simulink model "flightSimulator"  (R2022a)
settings: Solver=VariableStepAuto  StartTime=0.0  StopTime=10.0  RelTol=1e-3
values from neighbouring files (symbols this model uses):
  g = 9.81    [LQRCalcs.m]    (also in cf_firstOrderStateMdl.m; init_parameters.m; main.m; parameters_buildingSimulink.m)
  Gamma = [cT, cT, cT, cT ... (first row only)    [init_parameters.m]    (also in parameters_buildingSimulink.m; parameters_init.m; parameters_init2.m; parameters_init____CodeToImplementLater.m)
  GammaInv = inv(Gamma)    [init_parameters.m]    (also in parameters_buildingSimulink.m; parameters_init.m; parameters_init2.m)
  J = cat(2, [0 0 0]', J)    [LQRCalcs.m]    (also in init_parameters.m = diag([0.082, 0.0845, 0.1377]); main.m = diag([0.082, 0.0845, 0.1377]); parameters_buildingSimulink.m = diag([0.082, 0.0845, 0.1377]); parameters_init.m = Crazyflie.J)
  k_motors = 1    [parameters_buildingSimulink.m]
  k_R = 8.81    [init_parameters.m]    (also in parameters_init____CodeToImplementLater.m)
  Kd_attitude = 0.01    [parameters_buildingSimulink.m]
  Kd_eta = 0    [init_parameters.m]
  Kp_attitude = 0.5    [parameters_buildingSimulink.m]
  Kp_eta = 0    [init_parameters.m]
  m = 0.003    [LQRCalcs.m]    (also in cf_firstOrderStateMdl.m; init_parameters.m = 4.34; main.m = 4.34; parameters_buildingSimulink.m = 4.34)
  XYZ_initial_condition = [0, 0, 0]'    [init_parameters.m]
undefined symbols (not defined in the file or in its folder): k_Omega
libraries: slpidlib x2, aerolibutil x2
settings Model: Creator=Drew Lab Computer 1  LastModifiedBy=Drew Lab Computer 1

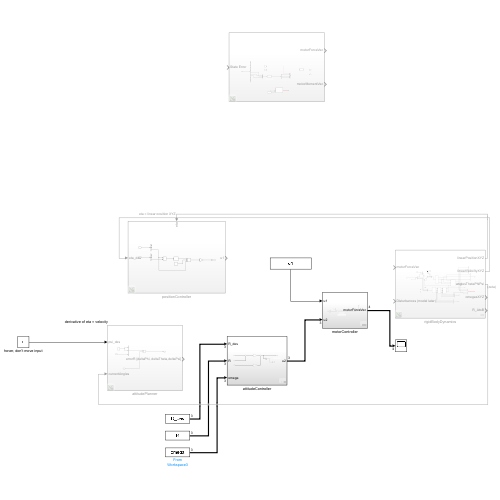
[thumbnail: Simulink's stored preview of the top-level diagram]
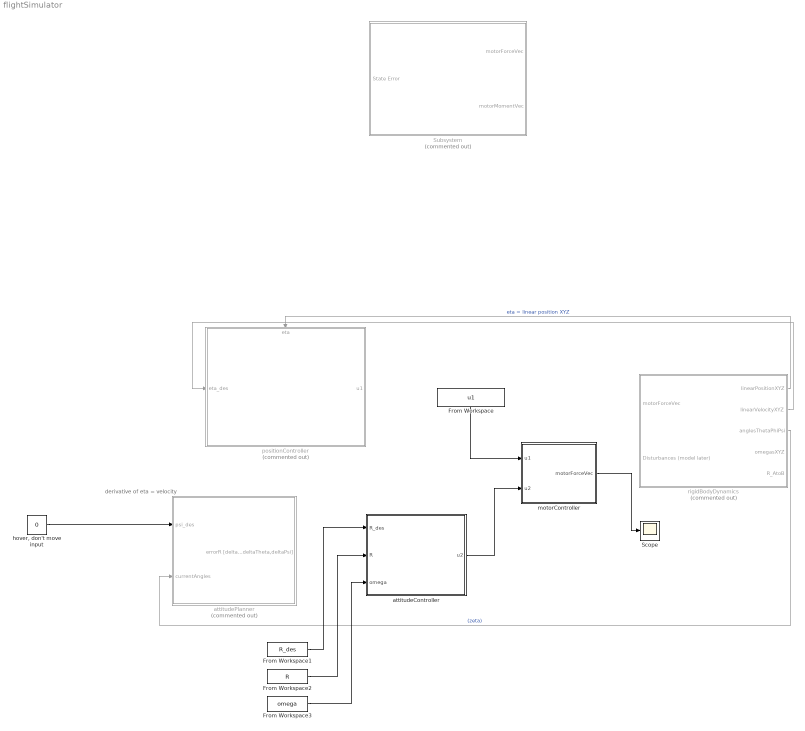
== system flightSimulator ==
  note: derivative of eta = velocity
  From Workspace : FromWorkspace  VariableName=u1
  From Workspace1 : FromWorkspace  VariableName=R_des
  From Workspace2 : FromWorkspace  VariableName=R
  From Workspace3 : FromWorkspace  VariableName=omega
  Scope : Scope
  Subsystem : Subsystem  Commented=on
  attitudeController : Subsystem
  attitudePlanner : Subsystem  Commented=on
  "hover, don't move input" : Constant  Value=0
  motorController : Subsystem
  positionController : Subsystem  Commented=on
      settings: PortSchema="{\"entries\":[{\"content\":{\"sides\":[{\"content\":{\"connectorIds\":[\"In1\"]},\"type\":\"ConnectorPlacement.EquallySpacedRectSide\",\"uuid\":\"de936069-44f0-4aa9-b4b1-7b3705576372\"},{\"content\":{\"connectorIds\":[\"Out1\"],\"side\":\"RIGHT\"},\"type\":\"ConnectorPlacement.EquallySpacedRectSide\",\"uuid\":\"f2caec36-291a-4389-af1f-a91b49b87c15\"},{\"content\":{\"connectorIds\":[\"In2\"],\"side\":\"TOP\"},\"type\":\"ConnectorPlacement.EquallySpacedRectSide\",\"uuid\":\"cd074ac1-2f19-4ea9-a351-803ac25dc689\"}]},\"type\":\"ConnectorPlacement.EquallySpacedConnector\",\"uuid\":\"58e30618-1523-4ed1-9bdc-0936c58338cb\"}],\"packageUris\":[\"http://schema.mathworks.com/mf0/Connector/R2020b\"],\"version\":\"1.0\"}"
  rigidBodyDynamics : Subsystem  Commented=on
  wires:
  rigidBodyDynamics/1(linearPositionXYZ) -> positionController/2(eta)  "eta = linear position XYZ"
  rigidBodyDynamics/3(anglesThetaPhiPsi) -> attitudePlanner/2(currentAngles)  "(zeta)"
  "hover, don't move input"/1 -> attitudePlanner/1(psi_des)
  rigidBodyDynamics/2(linearVelocityXYZ) -> positionController/1(eta_des)
  attitudeController/1(u2) -> motorController/2(u2)
  From Workspace/1 -> motorController/1(u1)
  From Workspace1/1 -> attitudeController/1(R_des)
  From Workspace2/1 -> attitudeController/2(R)
  From Workspace3/1 -> attitudeController/3(omega)
  motorController/1(motorForceVec) -> Scope/1

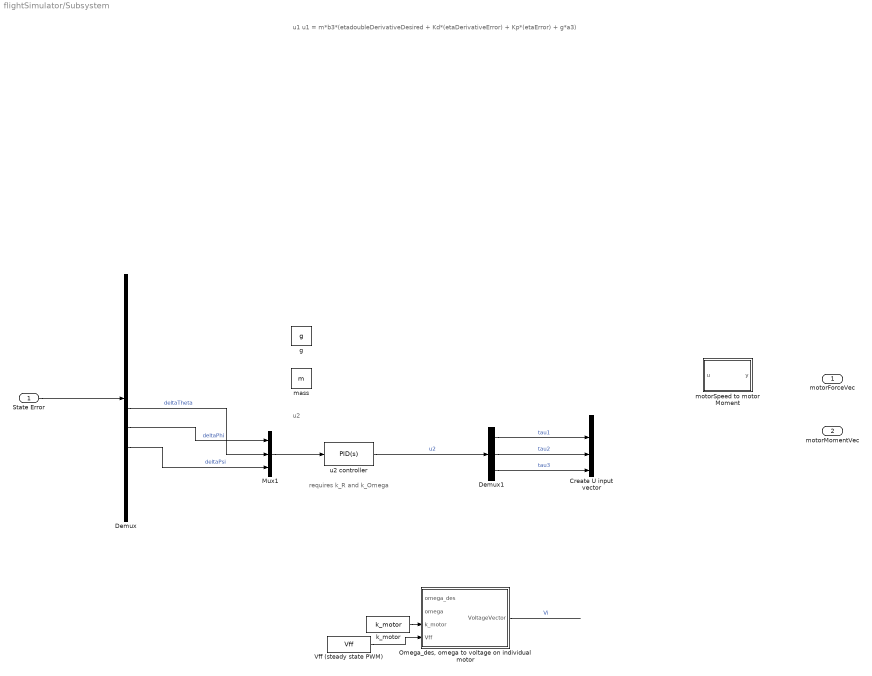
== system flightSimulator/Subsystem ==
  note: requires k_R and k_Omega
  note: u2
  note: u1
      | u1 = m*b3*(etadoubleDerivativeDesired + Kd*(etaDerivativeError) + Kp*(etaError) + g*a3)
  State Error : Inport
  Create U input vector : Mux
  Demux : Demux  Outputs=12
  Demux1 : Demux  Outputs=3
  Mux1 : Mux  Inputs=3
  "Omega_des, omega to voltage on individual motor" : MATLAB Function  TreatAsAtomicUnit=on
  Vff (steady state PWM) : FromWorkspace  VariableName=Vff
  g : Constant  Value=g
  k_motor : FromWorkspace  VariableName=k_motor
  mass : Constant  Value=m
  motorSpeed to motor Moment : MATLAB Function  TreatAsAtomicUnit=on
  u2 controller : slpidlib/PID Controller  Controller=PID  Form=Parallel  TimeDomain=Continuous-time  UseExternalTs=off  SampleTime=-1  IntegratorMethod=Forward Euler  FilterMethod=Forward Euler  ControllerParametersSource=internal  P=k_R  I=1  UseKiTs=off  D=k_Omega  N=100  UseFilter=on  TunerSelectOption=Transfer Function Based (PID Tuner App)  InitialConditionSource=internal  InitialConditionForIntegrator=0  InitialConditionForFilter=0  DifferentiatorICPrevScaledInput=0  ExternalReset=none  TrackingMode=off  Kt=1  LimitOutput=off  SatLimitsSource=internal  UpperSaturationLimit=inf  LowerSaturationLimit=-inf  LinearizeAsGain=on  AntiWindupMode=none  Kb=1  POutMin=[]  POutMax=[]  IOutMin=[]  IOutMax=[]  DOutMin=[]  DOutMax=[]  NOutMin=[]  NOutMax=[]  SumOutMin=[]  SumOutMax=[]  SaturationOutMin=[]  SaturationOutMax=[]  PParamMin=[]  PParamMax=[]  IParamMin=[]  IParamMax=[]  DParamMin=[]  DParamMax=[]  NParamMin=[]  NParamMax=[]  KbParamMin=[]  KbParamMax=[]  KtParamMin=[]  KtParamMax=[]  KbOutMin=[]  KbOutMax=[]  KtOutMin=[]  KtOutMax=[]  IntegratorOutMin=[]  IntegratorOutMax=[]  FilterOutMin=[]  FilterOutMax=[]  SumI1OutMin=[]  SumI1OutMax=[]  SumI2OutMin=[]  SumI2OutMax=[]  SumI3OutMin=[]  SumI3OutMax=[]  SumI4OutMin=[]  SumI4OutMax=[]  SumDOutMin=[]  SumDOutMax=[]  DifferentiatorOutMin=[]  DifferentiatorOutMax=[]  FilterDiffOutCoefMin=[]  FilterDiffOutCoefMax=[]  ReciprocalOutMin=[]  ReciprocalOutMax=[]  SumDenOutMin=[]  SumDenOutMax=[]  SumNumOutMin=[]  SumNumOutMax=[]  DivideOutMin=[]  DivideOutMax=[]  UdiffTsProdOutMin=[]  UdiffTsProdOutMax=[]  NTsProdOutMin=[]  NTsProdOutMax=[]  UintegralTsProdOutMin=[]  UintegralTsProdOutMax=[]  UngainTsProdOutMin=[]  UngainTsProdOutMax=[]  IntegratorContinuousStateAttributes=''  IntegratorStateMustResolveToSignalObject=off  IntegratorRTWStateStorageClass=Auto  FilterContinuousStateAttributes=''  FilterStateMustResolveToSignalObject=off  FilterRTWStateStorageClass=Auto  ParallelPVariant=InternalParameters  IdealPVariant=Disabled  IVariant=InternalParameters  DVariant=InternalParameters  IntegratorVariant=Continuous  SatVariant=Disabled  AWVariant=Passthrough  PCopyVariant=Disabled  TRVariant=Disabled  FdbkBlocksVariant=Forward  IdealPFdbkVariant=Disabled  SatFdbkVariant=Disabled  DerivativeFilterVariant=ContFilter  NVariant=InternalParameters  NCopyVariant=Disabled  FilterICVariant=InternalICsFilter  IntegratorICVariant=InternalICs  ExternalResetVariant=Disabled  TRSumVariant=Passthrough  SumFdbkVariant=Disabled  SumVariant=Sum_PID  TsampFilterVariant=InternalTs  TsampNgainVariant=Passthrough  TsampIntegralVariant=Passthrough  ExternalSaturationOutDataTypeStr=Inherit: Same as second input  aMode=0
  motorForceVec : Outport
  motorMomentVec : Outport  Port=2
  wires:
  "Omega_des, omega to voltage on individual motor"/1(VoltageVector) -> ?  "Vi"
  State Error/1 -> Demux/1
  Demux/8 -> Mux1/1  "deltaPhi"
  Demux/9 -> Mux1/3  "deltaPsi"
  k_motor/1 -> "Omega_des, omega to voltage on individual motor"/3(k_motor)
  Vff (steady state PWM)/1 -> "Omega_des, omega to voltage on individual motor"/4(Vff)
  Demux/7 -> Mux1/2  "deltaTheta"
  Mux1/1 -> u2 controller/1
  u2 controller/1 -> Demux1/1  "u2"
  ? -> Create U input vector/1  "thrustSum"
  Demux1/3 -> Create U input vector/4  "tau3"
  Demux1/2 -> Create U input vector/3  "tau2"
  Demux1/1 -> Create U input vector/2  "tau1"

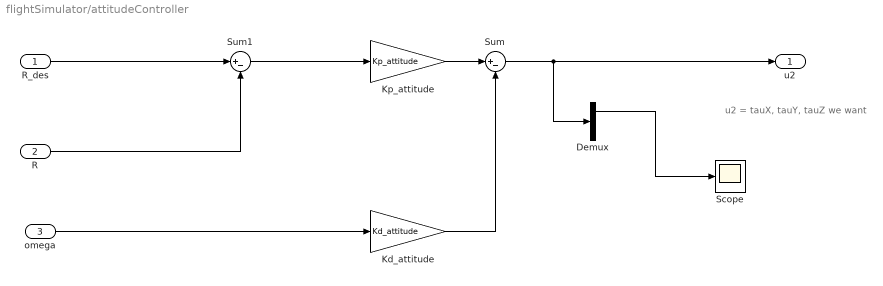
== system flightSimulator/attitudeController ==
  note: u2 = tauX, tauY, tauZ we want
  R_des : Inport
  R : Inport  Port=2
  omega : Inport  Port=3
  Demux : Demux  Outputs=3
  Kd_attitude : Gain  Gain=Kd_attitude
  Kp_attitude : Gain  Gain=Kp_attitude
  Scope : Scope
  Sum : Sum  Inputs=|+-
  Sum1 : Sum  Inputs=|+-
  u2 : Outport
  wires:
  Kp_attitude/1 -> Sum/1
  Kd_attitude/1 -> Sum/2
  Sum/1 -> Demux/1, u2/1
  R_des/1 -> Sum1/1
  R/1 -> Sum1/2
  Sum1/1 -> Kp_attitude/1
  omega/1 -> Kd_attitude/1
  Demux/1 -> Scope/1

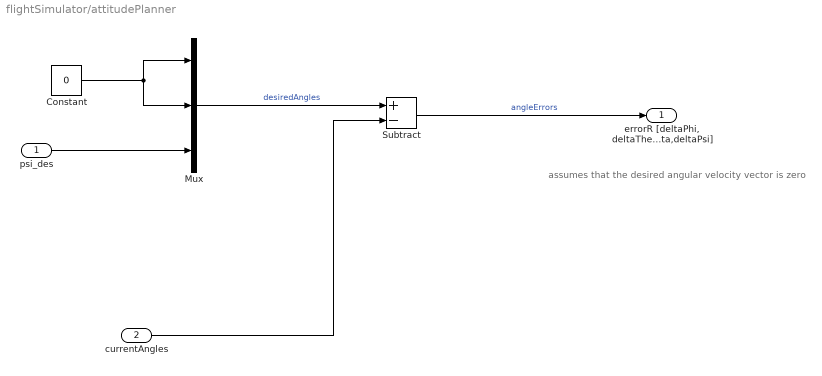
== system flightSimulator/attitudePlanner ==
  note: assumes that the desired angular velocity vector is zero
  psi_des : Inport
  currentAngles : Inport  Port=2
  Constant : Constant  Value=0
  Mux : Mux  Inputs=3
  Subtract : Sum  Inputs=+-
  "errorR [deltaPhi, deltaTheta,deltaPsi]" : Outport
  wires:
  psi_des/1 -> Mux/3
  Constant/1 -> Mux/1, Mux/2
  Mux/1 -> Subtract/1  "desiredAngles"
  Subtract/1 -> "errorR [deltaPhi, deltaTheta,deltaPsi]"/1  "angleErrors"
  currentAngles/1 -> Subtract/2

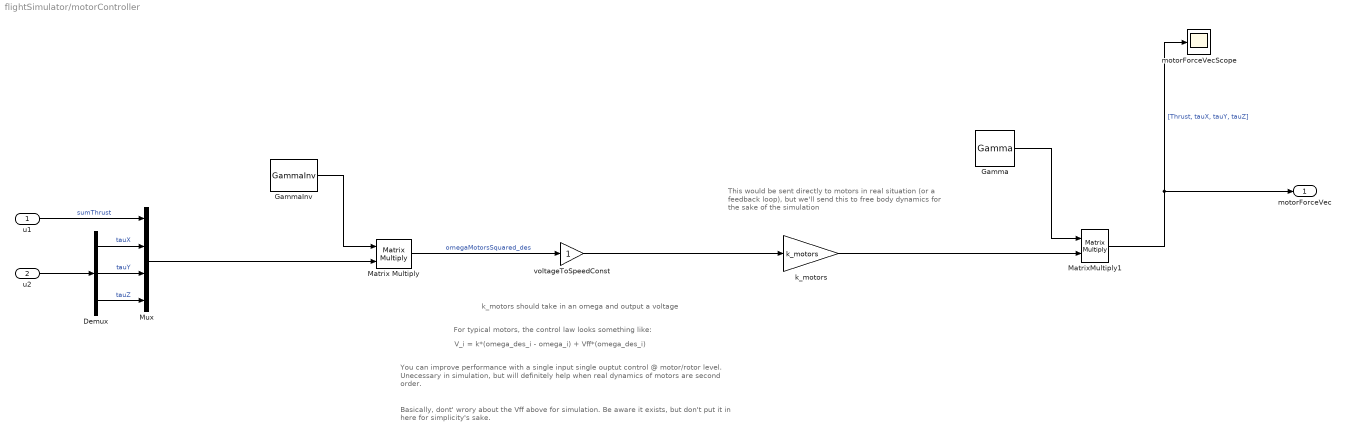
== system flightSimulator/motorController ==
  note: This would be sent directly to motors in real situation (or a feedback loop), but we'll send this to free body dynamics for the sake of the simulation
  note: k_motors should take in an omega and output a voltage
  note: Basically, dont' wrory about the Vff above for simulation. Be aware it exists, but don't put it in here for simplicity's sake.
  note: You can improve performance with a single input single ouptut control @ motor/rotor level. Unecessary in simulation, but will definitely help when real dynamics of motors are second order.
  note: V_i = k*(omega_des_i - omega_i) + Vff*(omega_des_i)
  note: For typical motors, the control law looks something like:
  u1 : Inport
  u2 : Inport  Port=2
  Demux : Demux  Outputs=3
  Gamma : Constant  Value=Gamma
  GammaInv : Constant  Value=GammaInv
  Matrix Multiply : Product  Multiplication=Matrix(*)
  MatrixMultiply1 : Product  Multiplication=Matrix(*)
  Mux : Mux
  k_motors : Gain  Gain=k_motors
  motorForceVecScope : Scope
  voltageToSpeedConst : Gain
  motorForceVec : Outport
  wires:
  u2/1 -> Demux/1
  u1/1 -> Mux/1  "sumThrust"
  Demux/2 -> Mux/3  "tauY"
  Demux/1 -> Mux/2  "tauX"
  Demux/3 -> Mux/4  "tauZ"
  Gamma/1 -> MatrixMultiply1/1
  MatrixMultiply1/1 -> motorForceVec/1, motorForceVecScope/1  "[Thrust, tauX, tauY, tauZ]"
  Mux/1 -> Matrix Multiply/2
  GammaInv/1 -> Matrix Multiply/1
  Matrix Multiply/1 -> voltageToSpeedConst/1  "omegaMotorsSquared_des"
  voltageToSpeedConst/1 -> k_motors/1
  k_motors/1 -> MatrixMultiply1/2

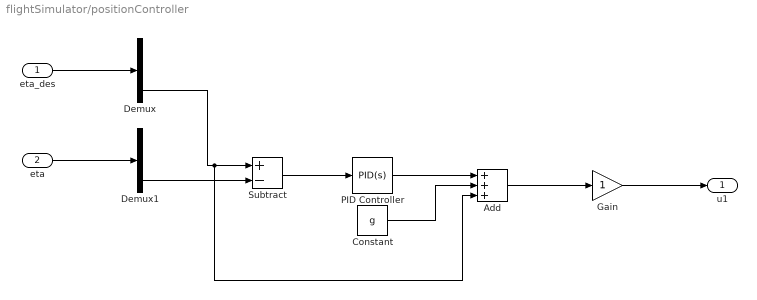
== system flightSimulator/positionController ==
  eta_des : Inport
  eta : Inport  Port=2
  Add : Sum  Inputs=+++
  Constant : Constant  Value=g
  Demux : Demux  Outputs=3
  Demux1 : Demux  Outputs=3
  Gain : Gain
  PID Controller : slpidlib/PID Controller  Controller=PID  Form=Parallel  TimeDomain=Continuous-time  UseExternalTs=off  SampleTime=-1  IntegratorMethod=Forward Euler  FilterMethod=Forward Euler  ControllerParametersSource=internal  P=Kp_eta  I=1  UseKiTs=off  D=Kd_eta  N=100  UseFilter=on  TunerSelectOption=Transfer Function Based (PID Tuner App)  InitialConditionSource=internal  InitialConditionForIntegrator=0  InitialConditionForFilter=0  DifferentiatorICPrevScaledInput=0  ExternalReset=none  TrackingMode=off  Kt=1  LimitOutput=off  SatLimitsSource=internal  UpperSaturationLimit=inf  LowerSaturationLimit=-inf  LinearizeAsGain=on  AntiWindupMode=none  Kb=1  POutMin=[]  POutMax=[]  IOutMin=[]  IOutMax=[]  DOutMin=[]  DOutMax=[]  NOutMin=[]  NOutMax=[]  SumOutMin=[]  SumOutMax=[]  SaturationOutMin=[]  SaturationOutMax=[]  PParamMin=[]  PParamMax=[]  IParamMin=[]  IParamMax=[]  DParamMin=[]  DParamMax=[]  NParamMin=[]  NParamMax=[]  KbParamMin=[]  KbParamMax=[]  KtParamMin=[]  KtParamMax=[]  KbOutMin=[]  KbOutMax=[]  KtOutMin=[]  KtOutMax=[]  IntegratorOutMin=[]  IntegratorOutMax=[]  FilterOutMin=[]  FilterOutMax=[]  SumI1OutMin=[]  SumI1OutMax=[]  SumI2OutMin=[]  SumI2OutMax=[]  SumI3OutMin=[]  SumI3OutMax=[]  SumI4OutMin=[]  SumI4OutMax=[]  SumDOutMin=[]  SumDOutMax=[]  DifferentiatorOutMin=[]  DifferentiatorOutMax=[]  FilterDiffOutCoefMin=[]  FilterDiffOutCoefMax=[]  ReciprocalOutMin=[]  ReciprocalOutMax=[]  SumDenOutMin=[]  SumDenOutMax=[]  SumNumOutMin=[]  SumNumOutMax=[]  DivideOutMin=[]  DivideOutMax=[]  UdiffTsProdOutMin=[]  UdiffTsProdOutMax=[]  NTsProdOutMin=[]  NTsProdOutMax=[]  UintegralTsProdOutMin=[]  UintegralTsProdOutMax=[]  UngainTsProdOutMin=[]  UngainTsProdOutMax=[]  IntegratorContinuousStateAttributes=''  IntegratorStateMustResolveToSignalObject=off  IntegratorRTWStateStorageClass=Auto  FilterContinuousStateAttributes=''  FilterStateMustResolveToSignalObject=off  FilterRTWStateStorageClass=Auto  ParallelPVariant=InternalParameters  IdealPVariant=Disabled  IVariant=InternalParameters  DVariant=InternalParameters  IntegratorVariant=Continuous  SatVariant=Disabled  AWVariant=Passthrough  PCopyVariant=Disabled  TRVariant=Disabled  FdbkBlocksVariant=Forward  IdealPFdbkVariant=Disabled  SatFdbkVariant=Disabled  DerivativeFilterVariant=ContFilter  NVariant=InternalParameters  NCopyVariant=Disabled  FilterICVariant=InternalICsFilter  IntegratorICVariant=InternalICs  ExternalResetVariant=Disabled  TRSumVariant=Passthrough  SumFdbkVariant=Disabled  SumVariant=Sum_PID  TsampFilterVariant=InternalTs  TsampNgainVariant=Passthrough  TsampIntegralVariant=Passthrough  ExternalSaturationOutDataTypeStr=Inherit: Same as second input  aMode=0
  Subtract : Sum  Inputs=+-
  u1 : Outport
  wires:
  eta_des/1 -> Demux/1
  Subtract/1 -> PID Controller/1
  eta/1 -> Demux1/1
  Demux/3 -> Add/3, Subtract/1
  Demux1/3 -> Subtract/2
  PID Controller/1 -> Add/1
  Constant/1 -> Add/2
  Add/1 -> Gain/1
  Gain/1 -> u1/1

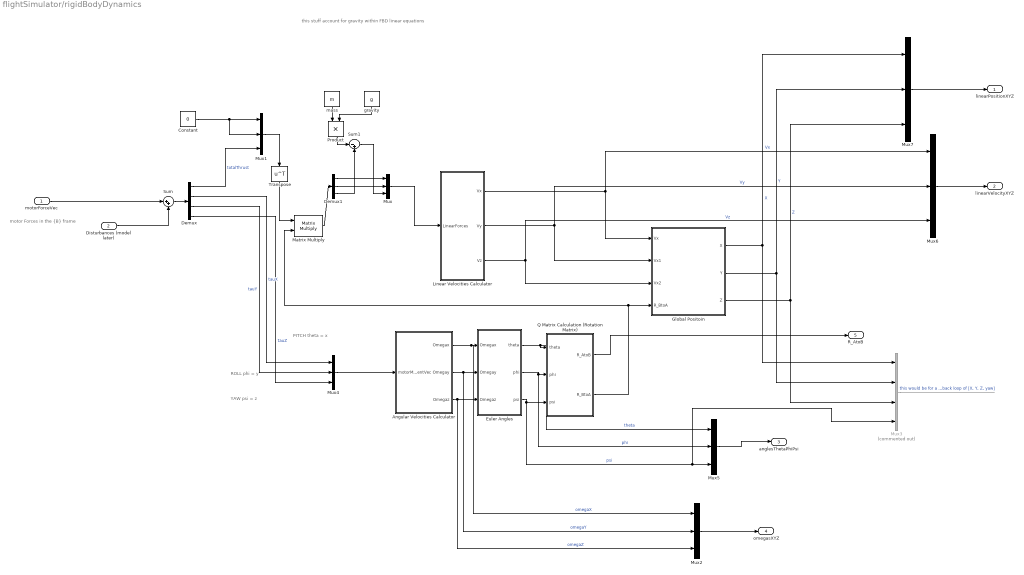
== system flightSimulator/rigidBodyDynamics ==
  note: YAW
      | psi = z
  note: ROLL
      | phi = y
  note: PITCH
      | theta = x
  note: this stuff account for gravity within FBD linear equations
  note: motor Forces in the {B} frame
  motorForceVec : Inport
  Disturbances (model later) : Inport  Port=2
  Angular Velocities Calculator : Subsystem
  Constant : Constant  Value=0
  Demux : Demux
  Demux1 : Demux  Outputs=3
  Euler Angles : Subsystem
  Global Positoin : Subsystem
  Linear Velocities Calculator : Subsystem
  Matrix Multiply : Product  Multiplication=Matrix(*)
  Mux{,1..2,4..7} (7 alike) : Mux  Inputs=3
  Mux3 : Mux  Commented=on
  Product : Product
  Q Matrix Calculation (Rotation Matrix) : Subsystem
  Sum : Sum  Inputs=|++
  Sum1 : Sum  Inputs=|-+
  Transpose : Math  Operator=transpose
  gravity : Constant  Value=g
  mass : Constant  Value=m
  linearPositionXYZ : Outport
  linearVelocityXYZ : Outport  Port=2
  anglesThetaPhiPsi : Outport  Port=3
  omegasXYZ : Outport  Port=4
  R_AtoB : Outport  Port=5
  wires:
  Transpose/1 -> Matrix Multiply/1
  Mux1/1 -> Transpose/1
  motorForceVec/1 -> Sum/1
  Disturbances (model later)/1 -> Sum/2
  Linear Velocities Calculator/1(Vx) -> Mux6/1, Global Positoin/1(Vx)  "Vx"
  Linear Velocities Calculator/2(Vy) -> Mux6/2, Global Positoin/2(Vx1)  "Vy"
  Linear Velocities Calculator/3(Vz) -> Mux6/3, Global Positoin/3(Vx2)  "Vz"
  Q Matrix Calculation (Rotation Matrix)/2(R_BtoA) -> Matrix Multiply/2, Global Positoin/4(R_BtoA)
  Mux4/1 -> Angular Velocities Calculator/1(motorMomentVec)
  Angular Velocities Calculator/3(Omegaz) -> Mux2/3, Euler Angles/3(Omegaz)  "omegaZ"
  Angular Velocities Calculator/2(Omegay) -> Mux2/2, Euler Angles/2(Omegay)  "omegaY"
  Angular Velocities Calculator/1(Omegax) -> Mux2/1, Euler Angles/1(Omegax)  "omegaX"
  Euler Angles/2(phi) -> Mux5/2, Q Matrix Calculation (Rotation Matrix)/2(phi)  "phi"
  Euler Angles/1(theta) -> Mux5/1, Q Matrix Calculation (Rotation Matrix)/1(theta)  "theta"
  Euler Angles/3(psi) -> Mux3/4, Mux5/3, Q Matrix Calculation (Rotation Matrix)/3(psi)  "psi"
  Mux/1 -> Linear Velocities Calculator/1(LinearForces)
  Product/1 -> Sum1/1
  Sum1/1 -> Mux/3
  mass/1 -> Product/1
  gravity/1 -> Product/2
  Global Positoin/3(Z) -> Mux7/3, Mux3/3  "Z"
  Global Positoin/2(Y) -> Mux7/2, Mux3/2  "Y"
  Global Positoin/1(X) -> Mux7/1, Mux3/1  "X"
  Mux3/1 -> ?  "this would be for a feedback loop of [X, Y, Z, yaw]"
  Sum/1 -> Demux/1
  Demux/1 -> Mux1/3  "totalThrust"
  Demux1/3 -> Sum1/2
  Demux1/2 -> Mux/2
  Demux1/1 -> Mux/1
  Demux/3 -> Mux4/2  "tauY"
  Demux/4 -> Mux4/3  "tauZ"
  Demux/2 -> Mux4/1  "tauX"
  Q Matrix Calculation (Rotation Matrix)/1(R_AtoB) -> R_AtoB/1
  Mux2/1 -> omegasXYZ/1
  Mux5/1 -> anglesThetaPhiPsi/1
  Mux7/1 -> linearPositionXYZ/1
  Mux6/1 -> linearVelocityXYZ/1
  Constant/1 -> Mux1/2, Mux1/1
  Matrix Multiply/1 -> Demux1/1

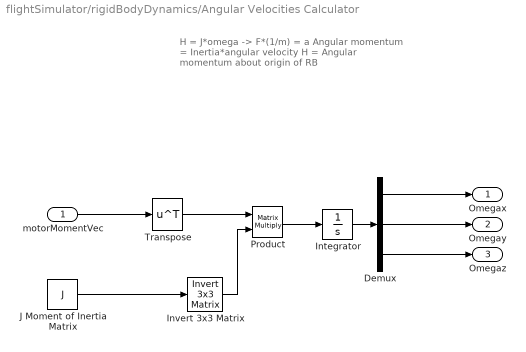
== system flightSimulator/rigidBodyDynamics/Angular Velocities Calculator ==
  note: H = J*omega -> F*(1/m) = a
      | Angular momentum = Inertia*angular velocity
      | H = Angular momentum about origin of RB
  motorMomentVec : Inport
  Demux : Demux  Outputs=3
  Integrator : Integrator
  Invert 3x3 Matrix : aerolibutil/Invert  3x3 Matrix
  J Moment of Inertia Matrix : Constant  Value=J
  Product : Product  Multiplication=Matrix(*)
  Transpose : Math  Operator=transpose
  Omegax : Outport
  Omegay : Outport  Port=2
  Omegaz : Outport  Port=3
  wires:
  Transpose/1 -> Product/1
  motorMomentVec/1 -> Transpose/1
  Demux/1 -> Omegax/1
  Demux/2 -> Omegay/1
  Demux/3 -> Omegaz/1
  Product/1 -> Integrator/1
  Integrator/1 -> Demux/1
  J Moment of Inertia Matrix/1 -> Invert 3x3 Matrix/1
  Invert 3x3 Matrix/1 -> Product/2

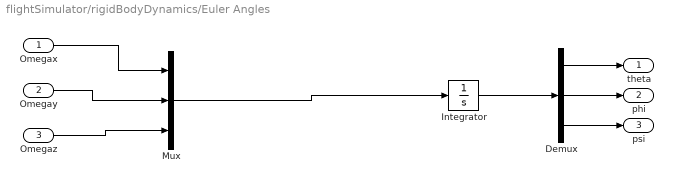
== system flightSimulator/rigidBodyDynamics/Euler Angles ==
  Omegax : Inport
  Omegay : Inport  Port=2
  Omegaz : Inport  Port=3
  Demux : Demux  Outputs=3
  Integrator : Integrator
  Mux : Mux  Inputs=3
  theta : Outport
  phi : Outport  Port=2
  psi : Outport  Port=3
  wires:
  Omegaz/1 -> Mux/3
  Omegay/1 -> Mux/2
  Omegax/1 -> Mux/1
  Integrator/1 -> Demux/1
  Demux/2 -> phi/1
  Demux/1 -> theta/1
  Demux/3 -> psi/1
  Mux/1 -> Integrator/1

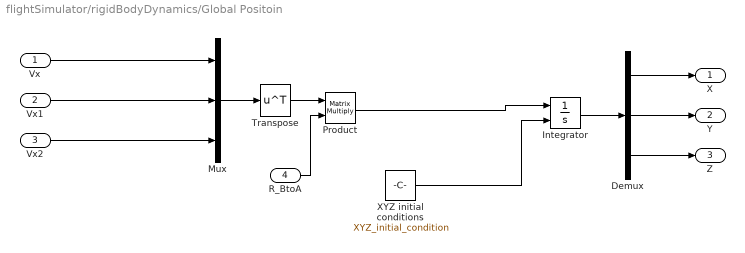
== system flightSimulator/rigidBodyDynamics/Global Positoin ==
  Vx : Inport
  Vx1 : Inport  Port=2
  Vx2 : Inport  Port=3
  R_BtoA : Inport  Port=4
  Demux : Demux  Outputs=3
  Integrator : Integrator  InitialConditionSource=external
  Mux : Mux  Inputs=3
  Product : Product  Multiplication=Matrix(*)
  Transpose : Math  Operator=transpose
  XYZ initial conditions : Constant  Value=XYZ_initial_condition
  X : Outport
  Y : Outport  Port=2
  Z : Outport  Port=3
  wires:
  Mux/1 -> Transpose/1
  Transpose/1 -> Product/1
  XYZ initial conditions/1 -> Integrator/2
  Product/1 -> Integrator/1
  Integrator/1 -> Demux/1
  Demux/2 -> Y/1
  Demux/1 -> X/1
  Demux/3 -> Z/1
  Vx2/1 -> Mux/3
  Vx1/1 -> Mux/2
  Vx/1 -> Mux/1
  R_BtoA/1 -> Product/2

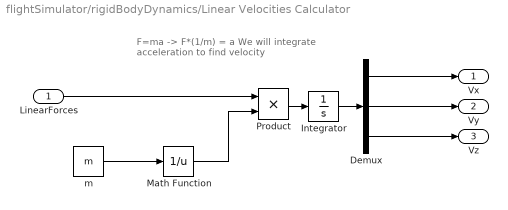
== system flightSimulator/rigidBodyDynamics/Linear Velocities Calculator ==
  note: F=ma -> F*(1/m) = a
      | We will integrate acceleration to find velocity
  LinearForces : Inport
  Demux : Demux  Outputs=3
  Integrator : Integrator
  Math Function : Math  Operator=reciprocal  SignedPower=on
  Product : Product
  m : Constant  Value=m
  Vx : Outport
  Vy : Outport  Port=2
  Vz : Outport  Port=3
  wires:
  LinearForces/1 -> Product/1
  m/1 -> Math Function/1
  Math Function/1 -> Product/2
  Demux/1 -> Vx/1
  Demux/2 -> Vy/1
  Demux/3 -> Vz/1
  Product/1 -> Integrator/1
  Integrator/1 -> Demux/1

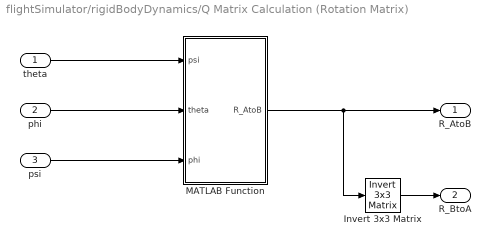
== system flightSimulator/rigidBodyDynamics/Q Matrix Calculation (Rotation Matrix) ==
  theta : Inport
  phi : Inport  Port=2
  psi : Inport  Port=3
  Invert 3x3 Matrix : aerolibutil/Invert  3x3 Matrix
  MATLAB Function : MATLAB Function  TreatAsAtomicUnit=on
  R_AtoB : Outport
  R_BtoA : Outport  Port=2
  wires:
  MATLAB Function/1(R_AtoB) -> Invert 3x3 Matrix/1, R_AtoB/1
  phi/1 -> MATLAB Function/2(theta)
  psi/1 -> MATLAB Function/3(phi)
  theta/1 -> MATLAB Function/1(psi)
  Invert 3x3 Matrix/1 -> R_BtoA/1

== matlab function flightSimulator/Subsystem/motorSpeed to motor Moment ==
  data: u input; y output
function y = fcn(u)

y = u;

== matlab function flightSimulator/rigidBodyDynamics/Q Matrix Calculation (Rotation Matrix)/MATLAB Function ==
  data: psi input; R_AtoB output; theta input; phi input
function R_AtoB = fcn(psi, theta, phi)

% R_AtoB = ...
%     [cos(psi)   -sin(psi) del_theta*cos(psi)+del_phi*sin(psi);
%      sin(psi),   cos(psi) del_theta*sin(psi)-del_phi*cos(psi);
%      -del_theta -del_phi 1;];

C_psi = cos(psi);
S_psi = sin(psi);
C_phi = cos(phi);
S_phi = sin(phi);
C_theta = cos(theta);
S_theta = sin(theta);
R_AtoB = ...
    [C_psi*C_theta-S_phi*S_psi*S_theta, -C_phi*S_phi, C_psi*S_theta+C_theta*S_phi*S_psi;
    C_theta*S_psi+C_psi*S_phi*S_theta, C_phi*C_psi, S_psi*S_theta-C_psi*C_theta*S_phi;
    -C_phi*S_theta, S_phi, C_phi*C_theta;];
%     [cos(psi)*cos(theta)-sin(phi)*sin(psi)*sin(theta), -cos(phi)*sin(psi), cos(phi)*sin(theta), cos(theta)*sin(phi)*sin(psi);
%     cos(theta)*sin(psi)+cos(psi)*sin(phi)*sin(theta), cos(phi)*cos(psi), sin(psi)*sin(theta)-cos(psi)*cos(theta)*sin(phi);
%     -cos(phi)*sin(theta), sin(phi), cos(phi)*cos(theta);];

== matlab function flightSimulator/Subsystem/Omega_des, omega to voltage on individual motor ==
  data: omega_des input; VoltageVector output; omega input; k_motor input; Vff input
function VoltageVector = fcn(omega_des, omega, k_motor, Vff)
% omega_des = [omega1, omega2, omega3, omega4]
% omega = [omega1, omega2, omega3, omega4]
[r, c] = size(omega)
omegaLen = max([r, c]) % picks whatever direction omega is in 
for i=[1:omegaLen]
    VoltageVector(i) = k_motor.*(omega_des(i) - omega(i)) + Vff.*(omega_des(i));

    
end
VoltageVector = VoltageVector'; %Formats V as a column vector output
